simulink model "chap4_5sim"  (Simulink 5.1)
settings: Solver=ode45  StartTime=0.0  StopTime=10  RelTol=1e-3
settings Model: LastModifiedBy=liu  ExtModeTrigMode=oneshot  ExtModeArmWhenConnect=off  LimitDataPoints=off  ProdHWDeviceType=Microprocessor

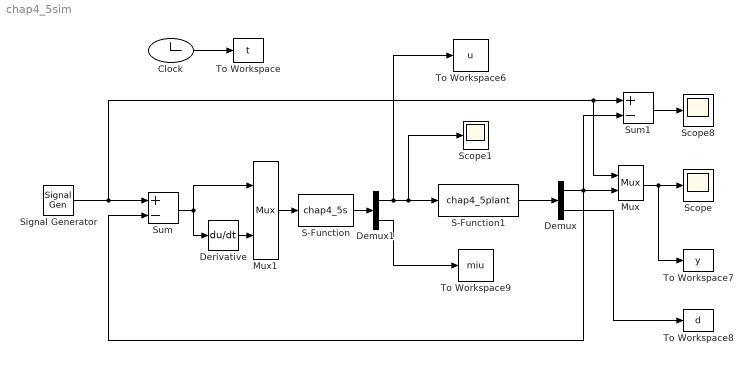
== system chap4_5sim ==
  Clock : Clock
  Demux : Demux  Outputs=2
  Demux1 : Demux  Outputs=2
  Derivative : Derivative
  Mux : Mux  Inputs=2
  Mux1 : Mux  Inputs=2
  S-Function : S-Function  FunctionName=chap4_5s
  S-Function1 : S-Function  FunctionName=chap4_5plant
  Scope : Scope
      settings: TimeRange=3  YMin=-1  YMax=1  MaxDataPoints=50000
  Scope1 : Scope
      settings: TimeRange=3  YMin=-1.25  YMax=1.25  MaxDataPoints=50000
  Scope8 : Scope
      settings: TimeRange=3  YMin=-0.0002  YMax=7.5e-005  MaxDataPoints=50000
  Signal Generator : SignalGenerator
  Sum : Sum  Inputs=+-  SaturateOnIntegerOverflow=on  InputSameDT=on
  Sum1 : Sum  Inputs=+-  SaturateOnIntegerOverflow=on  InputSameDT=on
  To Workspace : ToWorkspace  VariableName=t  SampleTime=-1  SaveFormat=Array
  To Workspace6 : ToWorkspace  VariableName=u  SampleTime=-1  SaveFormat=Array
  To Workspace7 : ToWorkspace  VariableName=y  SampleTime=-1  SaveFormat=Array
  To Workspace8 : ToWorkspace  VariableName=d  SampleTime=-1  SaveFormat=Array
  To Workspace9 : ToWorkspace  VariableName=miu  SampleTime=-1  SaveFormat=Array
  wires:
  Clock/1 -> To Workspace/1
  S-Function1/1 -> Demux/1
  Demux/2 -> To Workspace8/1
  Demux/1 -> Mux/2, Sum1/2, Sum/2
  Sum1/1 -> Scope8/1
  Mux/1 -> Scope/1, To Workspace7/1
  Mux1/1 -> S-Function/1
  Derivative/1 -> Mux1/2
  Sum/1 -> Mux1/1, Derivative/1
  Signal Generator/1 -> Sum/1, Sum1/1, Mux/1
  S-Function/1 -> Demux1/1
  Demux1/1 -> S-Function1/1, Scope1/1, To Workspace6/1
  Demux1/2 -> To Workspace9/1
